simulink model "model_tmp_1p"  (R2015b)
settings: Solver=ode15s  StartTime=0.0  StopTime=T_sim  FixedStep=dt  RelTol=1e-3
PreLoadFcn:
  | setup_tmp_1p;
InitFcn:
  | setup_tmp_1p;
values from neighbouring files (symbols this model uses):
  A_act = [-100 0 0 0 0 -100 0 0 0 0 -100 0 ... (16 elements, 4x4)]    [CD_spline.mat]    (also in CL_spline.mat; setup.m = -100*eye(4); setup_tmp_1p.m = -100*eye(4); setup_tmp_4p.m = -100*eye(4))
  A_Kite = 7    [CD_spline.mat]    (also in CL_spline.mat; setup.m = 10.18; setup_tmp_1p.m = 10.18; setup_tmp_4p.m = 10.18)
  A_prd = [0 0 0 -640 0 0 0 0 0 0 -640 0 ... (36 elements, 6x6)]    [CD_spline.mat]    (also in CL_spline.mat; setup.m = 1000 * A_M_aug; setup_tmp_1p.m = 1000 * A_M_aug; setup_tmp_4p.m = 1000 * A_M_aug)
  A_ref = [0 0 0 -10000 0 0 0 0 0 0 -10000 0 ... (36 elements, 6x6)]    [CD_spline.mat]    (also in CL_spline.mat; setup.m = zeros(6); setup_tmp_1p.m = zeros(6); setup_tmp_4p.m = zeros(6))
  A_t_ref_cl = [0 0 0 -0.64 0 0 0 0 0 0 -0.64 0 ... (36 elements, 6x6)]    [CD_spline.mat]    (also in CL_spline.mat; setup.m = A_t_ref; setup_tmp_1p.m = A_t_ref; setup_tmp_4p.m = A_t_ref)
  ASideRel = 0    [CD_spline.mat]    (also in CL_spline.mat; setup.m; setup_tmp_1p.m; setup_tmp_4p.m)
  B_act = [100 0 0 0 0 100 0 0 0 0 100 0 ... (16 elements, 4x4)]    [CD_spline.mat]    (also in CL_spline.mat; setup.m = 100*eye(4); setup_tmp_1p.m = 100*eye(4); setup_tmp_4p.m = 100*eye(4))
  B_ref = [0 0 0 10000 0 0 0 0 0 0 10000 0 ... (18 elements, 6x3)]    [CD_spline.mat]    (also in CL_spline.mat; setup.m = zeros(6,3); setup_tmp_1p.m = zeros(6,3); setup_tmp_4p.m = zeros(6,3))
  B_t_ref_cl = [0 0 0 0.64 0 0 0 0 0 0 0.64 0 ... (18 elements, 6x3)]    [CD_spline.mat]    (also in CL_spline.mat)
  Bpbl = [0 0 0 1 0 0 0 0 0 0 1 0 ... (18 elements, 6x3)]    [CD_spline.mat]    (also in CL_spline.mat; setup.m = [zeros(3); eye(3)]; setup_tmp_1p.m = [zeros(3); eye(3)]; setup_tmp_4p.m = [zeros(3); eye(3)])
  c0 = 614000    [CD_spline.mat]    (also in CL_spline.mat; setup.m; setup_tmp_1p.m; setup_tmp_4p.m)
  C_A = [0 0.3 -1e-06 1 -0.3 0 1e-06 1 0 -0.3 -1e-06 1 ... (16 elements, 4x4)]    [CD_spline.mat]    (also in CL_spline.mat; setup.m = [0, -R, 0, R; setup_tmp_1p.m = [0, -R, 0, R; setup_tmp_4p.m = [0, -R, 0, R)
  C_A_inv = [0 -1.66666666667 -1.23358113847e-17 1.66666666667 1.66666666667 2.46716227694e-17 -1.66666666667 0 -250000 250000 -250000 250000 ... (16 elements, 4x4)]    [CD_spline.mat]    (also in CL_spline.mat; setup.m = C_A \eye(4); setup_tmp_1p.m = C_A \eye(4); setup_tmp_4p.m = C_A \eye(4))
  C_D_Kite = 0.05    [CD_spline.mat]    (also in CL_spline.mat; setup.m = 0.005; setup_tmp_1p.m = 0.005; setup_tmp_4p.m = 0.005)
  C_L_Kite = 0.1    [CD_spline.mat]    (also in CL_spline.mat; setup.m = 0.01; setup_tmp_1p.m = 0.01; setup_tmp_4p.m = 0.01)
  CD_tether = 0.96    [CD_spline.mat]    (also in CL_spline.mat; setup.m; setup_tmp_1p.m; setup_tmp_4p.m)
  d0 = 473    [CD_spline.mat]    (also in CL_spline.mat; setup.m; setup_tmp_1p.m; setup_tmp_4p.m)
  d_tether = 0.004    [CD_spline.mat]    (also in CL_spline.mat; setup.m; setup_tmp_1p.m; setup_tmp_4p.m)
  delta_dead = 0.5    [CD_spline.mat]    (also in CL_spline.mat; setup.m; setup_tmp_1p.m; setup_tmp_4p.m)
  e_0 = 0.01    [CD_spline.mat]    (also in CL_spline.mat; setup.m; setup_tmp_1p.m; setup_tmp_4p.m)
  epsilon = 0.6    [CD_spline.mat]    (also in CL_spline.mat; setup.m; setup_tmp_1p.m; setup_tmp_4p.m)
  eta_init = [0 0 0]    [CD_spline.mat]    (also in CL_spline.mat; setup.m = zeros(3,1); setup_tmp_1p.m = zeros(3,1); setup_tmp_4p.m = zeros(3,1))
  g = 9.81    [CD_spline.mat]    (also in CL_spline.mat; setup.m; setup_tmp_1p.m; setup_tmp_4p.m)
  g_vec = [0 0 9.81]    [CD_spline.mat]    (also in CL_spline.mat; setup.m = [0;0;9.81]; setup_tmp_1p.m = [0;0;9.81]; setup_tmp_4p.m = [0;0;9.81])
  Gamma_ad = 100    [CD_spline.mat]    (also in CL_spline.mat; setup.m = 100;100; setup_tmp_1p.m = 100;100; setup_tmp_4p.m = 100;100)
  Gamma_pred = 100    [CD_spline.mat]    (also in CL_spline.mat; setup.m; setup_tmp_1p.m; setup_tmp_4p.m)
  J = [0.018  0  0; 0  0.018  0; 0  0  0.009]    [CD_spline.mat]    (also in CL_spline.mat; setup.m = diag([Ixx, Iyy, Izz]); setup_tmp_1p.m = diag([Ixx, Iyy, Izz]); setup_tmp_4p.m = diag([Ixx, Iyy, Izz]))
  Jinv = [55.5555555556  0  0; 0  55.5555555556  0; 0  0  111.111111111]    [CD_spline.mat]    (also in CL_spline.mat; setup.m = J \ eye(3); setup_tmp_1p.m = J \ eye(3); setup_tmp_4p.m = J \ eye(3))
  k_e_eta = 10000    [CD_spline.mat]    (also in CL_spline.mat; setup.m; setup_tmp_1p.m; setup_tmp_4p.m)
  k_e_eta_dot = 400    [CD_spline.mat]    (also in CL_spline.mat; setup.m; setup_tmp_1p.m; setup_tmp_4p.m)
  k_e_eta_I = 1    [CD_spline.mat]    (also in CL_spline.mat; setup.m; setup_tmp_1p.m; setup_tmp_4p.m)
  K_i_t = [10  0  0; 0  10  0; 0  0  10]    [CD_spline.mat]    (also in CL_spline.mat; setup.m = 10*eye(3); setup_tmp_1p.m = 10*eye(3); setup_tmp_4p.m = 10*eye(3))
  K_v_t = [1.6  0  0; 0  1.6  0; 0  0  1.6]    [CD_spline.mat]    (also in CL_spline.mat; setup.m = 2*omega_0_trans*zeta_0_trans*eye(3); setup_tmp_1p.m = 2*omega_0_trans*zeta_0_trans*eye(3); setup_tmp_4p.m = 2*omega_0_trans*zeta_0_trans*eye(3))
  K_x_t = [0.64  0  0; 0  0.64  0; 0  0  0.64]    [CD_spline.mat]    (also in CL_spline.mat; setup.m = omega_0_trans^2*eye(3); setup_tmp_1p.m = omega_0_trans^2*eye(3); setup_tmp_4p.m = omega_0_trans^2*eye(3))
  l_s0 = 1    [CD_spline.mat]    (also in CL_spline.mat; setup.m = 1.42857142857; setup_tmp_1p.m = 1.42857142857; setup_tmp_4p.m = 2)
  m_kite = 7    [CD_spline.mat]    (also in CL_spline.mat; setup.m; setup_tmp_1p.m = 5;7; setup_tmp_4p.m = 6.21)
  m_p = 0.013    [CD_spline.mat]    (also in CL_spline.mat; setup.m = 0.0185714285714; setup_tmp_1p.m = 0.0185714285714; setup_tmp_4p.m = 0.026)
  m_uav = 3    [CD_spline.mat]    (also in CL_spline.mat; setup.m; setup_tmp_1p.m; setup_tmp_4p.m)
  n = 10    [CD_spline.mat]    (also in CL_spline.mat; setup.m; setup_tmp_1p.m; setup_tmp_4p.m)
  omega_init = [0 0 0]    [CD_spline.mat]    (also in CL_spline.mat; setup.m = zeros(3,1); setup_tmp_1p.m = zeros(3,1); setup_tmp_4p.m = zeros(3,1))
  p_init = [0 0 1 0 0 2 0 0 3 0 0 4 ... (30 elements, 30x1)]    [CD_spline.mat]    (also in CL_spline.mat; setup.m = zeros(3*n,1); setup_tmp_1p.m = zeros(3*n,1); setup_tmp_4p.m = zeros(3*n,1))
  P_prd = [712.5 0 0 156.25 0 0 0 712.5 0 0 156.25 0 ... (36 elements, 6x6)]    [CD_spline.mat]    (also in CL_spline.mat; setup.m = 1000 * P_tref; setup_tmp_1p.m = 1000 * P_tref; setup_tmp_4p.m = 1000 * P_tref)
  P_tref = [0.7125 0 0 0.15625 0 0 0 0.7125 0 0 0.15625 0 ... (36 elements, 6x6)]    [CD_spline.mat]    (also in CL_spline.mat; setup.m = lyap(A_M_aug', Q); setup_tmp_1p.m = lyap(A_M_aug', Q); setup_tmp_4p.m = lyap(A_M_aug', Q))
  rho_air = 1.225    [CD_spline.mat]    (also in CL_spline.mat; setup.m; setup_tmp_1p.m; setup_tmp_4p.m)
  rho_t = 0.013    [CD_spline.mat]    (also in CL_spline.mat; setup.m; setup_tmp_1p.m; setup_tmp_4p.m)
  sample_log = 0.01    [CD_spline.mat]    (also in CL_spline.mat; setup.m; setup_tmp_1p.m; setup_tmp_4p.m)
  t0 = 1    [CD_spline.mat]    (also in CL_spline.mat; setup.m; setup_tmp_1p.m; setup_tmp_4p.m)
  t1 = 3    [CD_spline.mat]    (also in CL_spline.mat; setup.m; setup_tmp_1p.m; setup_tmp_4p.m)
  T_launch = 40    [CD_spline.mat]    (also in CL_spline.mat; setup.m; setup_tmp_1p.m; setup_tmp_4p.m)
  Theta_max = 60    [CD_spline.mat]    (also in CL_spline.mat; setup.m; setup_tmp_1p.m; setup_tmp_4p.m)
  Thrust_Max = 80    [CD_spline.mat]    (also in CL_spline.mat; setup.m; setup_tmp_1p.m = 100; setup_tmp_4p.m = 1000000000)
  Tx = 10    [CD_spline.mat]    (also in CL_spline.mat; setup.m; setup_tmp_1p.m; setup_tmp_4p.m)
  Ty = 10    [CD_spline.mat]    (also in CL_spline.mat; setup.m; setup_tmp_1p.m; setup_tmp_4p.m)
  Tz = 10    [CD_spline.mat]    (also in CL_spline.mat; setup.m; setup_tmp_1p.m; setup_tmp_4p.m)
  v_w_vec = [1 1 1]    [CD_spline.mat]    (also in CL_spline.mat; setup.m = [1;0;0]; setup_tmp_1p.m = [1;0;0]; setup_tmp_4p.m = [1;0;0])
  x0num = 0    [CD_spline.mat]    (also in CL_spline.mat; polynomial_trajectory.m = double( solutions_x.x0 ))
  x1num = 0    [CD_spline.mat]    (also in CL_spline.mat; polynomial_trajectory.m = double( solutions_x.x1 ))
  x2num = 0    [CD_spline.mat]    (also in CL_spline.mat; polynomial_trajectory.m = double( solutions_x.x2 ))
  x3num = 0.05    [CD_spline.mat]    (also in CL_spline.mat; polynomial_trajectory.m = double( solutions_x.x3 ))
  x4num = -0.0075    [CD_spline.mat]    (also in CL_spline.mat; polynomial_trajectory.m = double( solutions_x.x4 ))
  x5num = 0.0003    [CD_spline.mat]    (also in CL_spline.mat; polynomial_trajectory.m = double( solutions_x.x5 ))
  x_drone_init = [0 0 10]    [CD_spline.mat]    (also in CL_spline.mat; setup.m = p_init(3*n-2:3*n); setup_KiteModel_4points.m = pos_UAV_init; setup_tmp_1p.m = p_init(3*n-2:3*n))
  xT = 5    [CD_spline.mat]    (also in CL_spline.mat; setup.m; setup_tmp_1p.m = 10; setup_tmp_4p.m = 10)
  y0num = 0    [CD_spline.mat]    (also in CL_spline.mat; polynomial_trajectory.m = double( solutions_y.y0 ))
  y1num = 0    [CD_spline.mat]    (also in CL_spline.mat; polynomial_trajectory.m = double( solutions_y.y1 ))
  y2num = 0    [CD_spline.mat]    (also in CL_spline.mat; polynomial_trajectory.m = double( solutions_y.y2 ))
  y3num = 0.1    [CD_spline.mat]    (also in CL_spline.mat; polynomial_trajectory.m = double( solutions_y.y3 ))
  y4num = -0.015    [CD_spline.mat]    (also in CL_spline.mat; polynomial_trajectory.m = double( solutions_y.y4 ))
  y5num = 0.0006    [CD_spline.mat]    (also in CL_spline.mat; polynomial_trajectory.m = double( solutions_y.y5 ))
  yT = 10    [CD_spline.mat]    (also in CL_spline.mat; setup.m; setup_tmp_1p.m = 0; setup_tmp_4p.m = 0)
  z0num = 10    [CD_spline.mat]    (also in CL_spline.mat; polynomial_trajectory.m = double( solutions_z.z0 ))
  z1num = 0    [CD_spline.mat]    (also in CL_spline.mat; polynomial_trajectory.m = double( solutions_z.z1 ))
  z2num = 0    [CD_spline.mat]    (also in CL_spline.mat; polynomial_trajectory.m = double( solutions_z.z2 ))
  z3num = 0.4    [CD_spline.mat]    (also in CL_spline.mat; polynomial_trajectory.m = double( solutions_z.z3 ))
  z4num = -0.06    [CD_spline.mat]    (also in CL_spline.mat; polynomial_trajectory.m = double( solutions_z.z4 ))
  z5num = 0.0024    [CD_spline.mat]    (also in CL_spline.mat; polynomial_trajectory.m = double( solutions_z.z5 ))
  zT = 50    [CD_spline.mat]    (also in CL_spline.mat; setup.m; setup_tmp_1p.m; setup_tmp_4p.m)
libraries: simulink x1
(part 2 of 2)

== system model_tmp_1p/Controller/Outer_Loop_Position/Adaptive_Augmentation/Proj(Theta_hat, GammaY)_1column ==
  note: Ref.: Lavretsky, Robust and Adaptive Control, p. 329
      | Lecure Notes Nonlinear and Adaptive Control, TU Munich, FSD, SS2014, Robustness Modifications
  Theta_hat : Inport
  Theta_dot : Inport  Port=2
  Mux : Mux  Inputs=3
  Proj(Theta,Theta_dot) : MATLAB Function  TreatAsAtomicUnit=on
  Reshape1 : Reshape  OutputDimensionality=Row vector (2-D)
  Reshape2 : Reshape  OutputDimensionality=Row vector (2-D)
  To Workspace1 : ToWorkspace  VariableName=proj_flat  SaveFormat=Timeseries  SampleTime=sample_log
      settings: Save2DSignal=2-D array (concatenate along first dimension)
  To Workspace2 : ToWorkspace  VariableName=Theta_dot_save  SampleTime=sample_log
      settings: Save2DSignal=2-D array (concatenate along first dimension)
  To Workspace3 : ToWorkspace  VariableName=orthogonal_part  SampleTime=sample_log
      settings: Save2DSignal=2-D array (concatenate along first dimension)
  calculate_f : MATLAB Function  TreatAsAtomicUnit=on
  calculate_gradf : MATLAB Function  TreatAsAtomicUnit=on
  max_allowable_bound : Constant  Value=Theta_max
  projection_tolerance : Constant  Value=epsilon
  Theta_hat_dot : Outport
  wires:
  Proj(Theta,Theta_dot)/2(Theta_hat_dot_) -> Reshape1/1, Theta_hat_dot/1
  Proj(Theta,Theta_dot)/1(flag) -> Mux/2
  Proj(Theta,Theta_dot)/3(direction) -> Mux/3
  Mux/1 -> To Workspace1/1
  calculate_gradf/1(gradf) -> Proj(Theta,Theta_dot)/2(gradf)
  Theta_hat/1 -> calculate_gradf/1(theta_hat), calculate_f/1(theta_hat)
  projection_tolerance/1 -> calculate_f/3(epsilon), calculate_gradf/3(epsilon)
  max_allowable_bound/1 -> calculate_f/2(Theta_max), calculate_gradf/2(Theta_max)
  Theta_dot/1 -> Proj(Theta,Theta_dot)/3(Theta_dot)
  calculate_f/1(f) -> Mux/1, Proj(Theta,Theta_dot)/1(f)
  Reshape1/1 -> To Workspace2/1
  Proj(Theta,Theta_dot)/4(orthogonal_part) -> Reshape2/1
  Reshape2/1 -> To Workspace3/1

== system model_tmp_1p/Controller/Outer_Loop_Position/Adaptive_Augmentation/Proj(Theta_hat, GammaY)_multicolumns ==
  note: Ref.: Lavretsky, Robust and Adaptive Control, p. 329
      | Lecure Notes Nonlinear and Adaptive Control, TU Munich, FSD, SS2014, Robustness Modifications
  Theta_hat : Inport
  Theta_dot : Inport  Port=2
  MATLAB Function : MATLAB Function  TreatAsAtomicUnit=on
  Matrix Concatenate : Concatenate  NumInputs=3  Mode=Multidimensional array
  Projection_Input_1 : Subsystem
  Projection_Input_2 : Subsystem
  Projection_Input_3 : Subsystem
  Theta_hat_dot : Outport
  wires:
  Theta_hat/1 -> MATLAB Function/1(Theta_hat)
  Theta_dot/1 -> MATLAB Function/2(Theta_hat_dot)
  Projection_Input_1/1(Out1) -> Matrix Concatenate/1
  MATLAB Function/1(Theta_hat_1) -> Projection_Input_1/1(In1)
  MATLAB Function/2(Theta_hat_dot_1) -> Projection_Input_1/2(In2)
  MATLAB Function/3(Theta_hat_2) -> Projection_Input_2/1(In1)
  MATLAB Function/4(Theta_hat_dot_2) -> Projection_Input_2/2(In2)
  MATLAB Function/6(Theta_hat_dot_3) -> Projection_Input_3/2(In2)
  MATLAB Function/5(Theta_hat_3) -> Projection_Input_3/1(In1)
  Projection_Input_2/1(Out1) -> Matrix Concatenate/2
  Projection_Input_3/1(Out1) -> Matrix Concatenate/3
  Matrix Concatenate/1 -> Theta_hat_dot/1

== system model_tmp_1p/Controller/Outer_Loop_Position/Adaptive_Augmentation/Smooth_Deadzone_MRAC ==
  note: Ref.: Lavretsky, Robust and Adaptive Control, p. 319
  e : Inport
  Dead_Zone_Mod1 : Constant  Value=delta_dead
  Dead_Zone_Mod2 : Constant  Value=e_0
  Dot Product : DotProduct  InputSameDT=on  OutDataTypeStr=Inherit: Inherit via internal rule
  Mux : Mux  Inputs=2
  Sqrt : Sqrt  SaturateOnIntegerOverflow=on
  To Workspace8 : ToWorkspace  VariableName=e_ref_mu  SaveFormat=Timeseries  SampleTime=sample_log
      settings: Save2DSignal=2-D array (concatenate along first dimension)
  smooth_deadzone : MATLAB Function  TreatAsAtomicUnit=on
  mu_dead : Outport
  wires:
  e/1 -> Dot Product/1, Dot Product/2
  Dead_Zone_Mod1/1 -> smooth_deadzone/2(delta_dead)
  Dead_Zone_Mod2/1 -> smooth_deadzone/3(e_0)
  Dot Product/1 -> Sqrt/1
  Sqrt/1 -> Mux/1, smooth_deadzone/1(e_norm)
  smooth_deadzone/1(mu_dead) -> Mux/2, mu_dead/1
  Mux/1 -> To Workspace8/1

== system model_tmp_1p/Controller/Outer_Loop_Position/Adaptive_Augmentation/Smooth_Deadzone_PMRAC ==
  note: Ref.: Lavretsky, Robust and Adaptive Control, p. 319
  e : Inport
  Dead_Zone_Mod1 : Constant  Value=delta_dead
  Dead_Zone_Mod2 : Constant  Value=e_0
  Dot Product : DotProduct  InputSameDT=on  OutDataTypeStr=Inherit: Inherit via internal rule
  Mux1 : Mux  Inputs=2
  Sqrt : Sqrt  SaturateOnIntegerOverflow=on
  To Workspace1 : ToWorkspace  VariableName=e_pref_mu  SaveFormat=Timeseries  SampleTime=sample_log
      settings: Save2DSignal=2-D array (concatenate along first dimension)
  smooth_deadzone : MATLAB Function  TreatAsAtomicUnit=on
  mu_dead : Outport
  wires:
  Dot Product/1 -> Sqrt/1
  Dead_Zone_Mod2/1 -> smooth_deadzone/3(e_0)
  Dead_Zone_Mod1/1 -> smooth_deadzone/2(delta_dead)
  e/1 -> Dot Product/2, Dot Product/1
  Sqrt/1 -> Mux1/1, smooth_deadzone/1(e_norm)
  smooth_deadzone/1(mu_dead) -> Mux1/2, mu_dead/1
  Mux1/1 -> To Workspace1/1

== system model_tmp_1p/Plant/Tether_Kite_Tether_UAV_Dynamics_1P/First_order_lag_Actuator/Actuator ==
  Propeller_RPMs_cmd : Inport
  Add : Sum  Inputs=+-
  Gain : Gain  Gain=B_act  Multiplication=Matrix(K*u)
  Gain1 : Gain  Gain=A_act  Multiplication=Matrix(K*u)
  Integrator Limited1 : Integrator  InitialCondition=zeros(4,1)  LimitOutput=on  UpperSaturationLimit=Thrust_Max  LowerSaturationLimit=-Thrust_Max
  Output_Actuator : Gain  Gain=C_A  Multiplication=Matrix(K*u)
  Reaction_Deficit_Actuators : Scope
  Sum : Sum  Inputs=|++
  To Workspace1 : ToWorkspace  VariableName=prop_thrust_cmd  SaveFormat=Timeseries  SampleTime=sample_log
  To Workspace2 : ToWorkspace  VariableName=prop_thrust_real  SaveFormat=Timeseries  SampleTime=sample_log
  Thrust_Moments : Outport
  wires:
  Output_Actuator/1 -> Thrust_Moments/1
  Gain/1 -> Sum/1
  Gain1/1 -> Sum/2
  Sum/1 -> Integrator Limited1/1
  Propeller_RPMs_cmd/1 -> Add/1, To Workspace1/1, Gain/1
  Add/1 -> Reaction_Deficit_Actuators/1
  Integrator Limited1/1 -> Add/2, To Workspace2/1, Gain1/1, Output_Actuator/1

== system model_tmp_1p/Controller/Outer_Loop_Position/Adaptive_Augmentation/Proj(Theta_hat, GammaY)_multicolumns/Projection_Input_1 ==
  In1 : Inport
  In2 : Inport  Port=2
  Proj(Theta,Theta_dot) : MATLAB Function  TreatAsAtomicUnit=on
  calculate_f : MATLAB Function  TreatAsAtomicUnit=on
  calculate_gradf : MATLAB Function  TreatAsAtomicUnit=on
  max_allowable_bound : Constant  Value=Theta_max
  projection_tolerance : Constant  Value=epsilon
  Out1 : Outport
  wires:
  calculate_f/1(f) -> Proj(Theta,Theta_dot)/1(f)
  In2/1 -> Proj(Theta,Theta_dot)/3(Theta_dot)
  max_allowable_bound/1 -> calculate_f/2(Theta_max), calculate_gradf/2(Theta_max)
  projection_tolerance/1 -> calculate_f/3(epsilon), calculate_gradf/3(epsilon)
  In1/1 -> calculate_gradf/1(theta_hat), calculate_f/1(theta_hat)
  calculate_gradf/1(gradf) -> Proj(Theta,Theta_dot)/2(gradf)
  Proj(Theta,Theta_dot)/1(Theta_hat_dot_) -> Out1/1

== system model_tmp_1p/Controller/Outer_Loop_Position/Adaptive_Augmentation/Proj(Theta_hat, GammaY)_multicolumns/Projection_Input_2 ==
  In1 : Inport
  In2 : Inport  Port=2
  Proj(Theta,Theta_dot) : MATLAB Function  TreatAsAtomicUnit=on
  calculate_f : MATLAB Function  TreatAsAtomicUnit=on
  calculate_gradf : MATLAB Function  TreatAsAtomicUnit=on
  max_allowable_bound : Constant  Value=Theta_max
  projection_tolerance : Constant  Value=epsilon
  Out1 : Outport
  wires:
  calculate_f/1(f) -> Proj(Theta,Theta_dot)/1(f)
  In2/1 -> Proj(Theta,Theta_dot)/3(Theta_dot)
  max_allowable_bound/1 -> calculate_f/2(Theta_max), calculate_gradf/2(Theta_max)
  projection_tolerance/1 -> calculate_f/3(epsilon), calculate_gradf/3(epsilon)
  In1/1 -> calculate_gradf/1(theta_hat), calculate_f/1(theta_hat)
  calculate_gradf/1(gradf) -> Proj(Theta,Theta_dot)/2(gradf)
  Proj(Theta,Theta_dot)/1(Theta_hat_dot_) -> Out1/1

== system model_tmp_1p/Controller/Outer_Loop_Position/Adaptive_Augmentation/Proj(Theta_hat, GammaY)_multicolumns/Projection_Input_3 ==
  In1 : Inport
  In2 : Inport  Port=2
  Mux : Mux  Inputs=3
  Proj(Theta,Theta_dot) : MATLAB Function  TreatAsAtomicUnit=on
  Scope : Scope
  Scope1 : Scope
  To Workspace1 : ToWorkspace  VariableName=proj_flat  SaveFormat=Timeseries  SampleTime=sample_log
      settings: Save2DSignal=2-D array (concatenate along first dimension)
  calculate_f : MATLAB Function  TreatAsAtomicUnit=on
  calculate_gradf : MATLAB Function  TreatAsAtomicUnit=on
  max_allowable_bound : Constant  Value=Theta_max
  projection_tolerance : Constant  Value=epsilon
  Out1 : Outport
  wires:
  calculate_f/1(f) -> Mux/1, Proj(Theta,Theta_dot)/1(f)
  In2/1 -> Proj(Theta,Theta_dot)/3(Theta_dot)
  max_allowable_bound/1 -> calculate_f/2(Theta_max), calculate_gradf/2(Theta_max)
  projection_tolerance/1 -> calculate_f/3(epsilon), calculate_gradf/3(epsilon)
  In1/1 -> calculate_gradf/1(theta_hat), calculate_f/1(theta_hat)
  calculate_gradf/1(gradf) -> Proj(Theta,Theta_dot)/2(gradf)
  Proj(Theta,Theta_dot)/2(Theta_hat_dot_) -> Out1/1
  Mux/1 -> To Workspace1/1
  Proj(Theta,Theta_dot)/3(direction) -> Scope/1, Mux/3
  Proj(Theta,Theta_dot)/1(flag) -> Scope1/1, Mux/2

== matlab function model_tmp_1p/Controller/Inner_Loop_Attitude/Plant_Inversion_RD2/Plant_Inversion ==
  data: omega input; u_NDI output; eta input; eta_dot input; J input; nu_tot input
function u_NDI = fcn(omega, eta, eta_dot, J, nu_tot)
%#codegen
p = omega(1); 
q = omega(2); 
r = omega(3); 
Ix = J(1,1); 
Iy = J(2,2); 
Iz = J(3,3); 


cross_coupling = [ Iy*q*r - Iz*q*r
 Iz*p*r - Ix*p*r;
 Ix*p*q - Iy*p*q];

% T_inv = [1, sin(eta(1)) * tan(eta(2)), cos(eta(1)) * tan(eta(2)) ; 
% 0, cos(eta(1)), -sin(eta(1)); 
% 0, sin(eta(1))/cos(eta(2)), cos(eta(1))/cos(eta(2))] \ eye(3); 

T_inv = [1, 0, -sin(eta(2));
         0, cos(eta(1)), sin(eta(1))*cos(eta(2));
         0, -sin(eta(1)), cos(eta(1))*cos(eta(2))];
     
T_dot = eta_dot(1) * [0, cos(eta(1)) * tan(eta(2)), -sin(eta(1))*tan(eta(2)); 
                      0, -sin(eta(1)), -cos(eta(1));
                      0, cos(eta(1))/cos(eta(2)), -sin(eta(1))/cos(eta(2))]+...
        eta_dot(2) * [0, sin(eta(1))/cos(eta(2))^2, cos(eta(1))/cos(eta(2))^2; 
                       0, 0, 0; 
                       0, sin(eta(1))*sin(eta(2))/cos(eta(2))^2, cos(eta(1))*sin(eta(2))/cos(eta(2))^2];
                          
u_NDI = -cross_coupling + J * T_inv * ( -T_dot * omega + nu_tot);

== matlab function model_tmp_1p/Flight_Path_Planner/Reference_Dynamic_x1 ==
  data: t input; y_ref output; y0num parameter; y1num parameter; y2num parameter; y3num parameter; y4num parameter; y5num parameter; yT parameter; Ty parameter
function y_ref = fcn(t,y0num, y1num, y2num, y3num, y4num, y5num, yT,Ty )

if t >= Ty
    y_ref = yT;
else
    y_ref = y5num * t^5 + y4num * t^4 + y3num * t^3 + y2num * t^2 + y1num * t + y0num;
end

== matlab function model_tmp_1p/Flight_Path_Planner/Reference_Dynamic_x3 ==
  data: t input; x_ref output; x0num parameter; x1num parameter; x2num parameter; x3num parameter; x4num parameter; x5num parameter; Tx parameter; xT parameter
function x_ref = fcn(t,x0num, x1num, x2num, x3num, x4num, x5num, Tx,xT )

if t >= Tx
    x_ref = xT;
else
    x_ref = x5num * t^5 + x4num * t^4 + x3num * t^3 + x2num * t^2 + x1num * t + x0num;
end

== matlab function model_tmp_1p/Flight_Path_Planner2/Reference_Dynamic_x ==
  data: x_cmd input; x_ref input; x_ref_dot output; t0 parameter; t1 parameter
function x_ref_dot = fcn(x_cmd, x_ref, t0, t1)

% a0 = 1;
% a1 = 5;

x_ref_dot = [0,1;
                -t0, -t1]*x_ref + [0;t0] * x_cmd;

== matlab function model_tmp_1p/Controller/Inner_Loop_Attitude/estimate_eta_dot ==
  data: omega input; eta input; eta_dot output
function eta_dot  = fcn( omega, eta)
%#codegen

eta_dot = [1, sin(eta(1)) * tan(eta(2)), cos(eta(1)) * tan(eta(2)) ; 
0, cos(eta(1)), -sin(eta(1)); 
0, sin(eta(1))/cos(eta(2)), cos(eta(1))/cos(eta(2))] * omega;

== matlab function model_tmp_1p/Flight_Path_Planner/Reference_Dynamic_x2 ==
  data: t input; z_ref output; z0num parameter; z1num parameter; z2num parameter; z3num parameter; z4num parameter; z5num parameter; Tz parameter; zT parameter
function z_ref = fcn(t,z0num, z1num, z2num, z3num, z4num, z5num,Tz, zT)

if t >= Tz
    z_ref = zT;
else
    z_ref = z5num * t^5 + z4num * t^4 + z3num * t^3 + z2num * t^2 + z1num * t + z0num;
end

== matlab function model_tmp_1p/Controller/Outer_Loop_Position/Adaptive_Augmentation/Smooth_Deadzone_PMRAC/smooth_deadzone ==
  data: e_norm input; mu_dead output; delta_dead input; e_0 input
function mu_dead = fcn(e_norm, delta_dead, e_0)
%#codegen

mu_dead = max( 0, min( 1, (e_norm - delta_dead*e_0)/...
                          ( (1-delta_dead) * e_0) ) );

== matlab function model_tmp_1p/Controller/Outer_Loop_Position/Predictor_Model_Translational_Dynamics/Reference_Model_Position ==
  data: A_prd input; A_ref input; x_prd_dotdot output; B_ref input; x_cmd input; x_p input; x_prd input
function x_prd_dotdot  = fcn(A_prd,A_ref,B_ref, x_cmd,x_p,x_prd)

    x_prd_dotdot = A_prd * (x_prd - x_p) + A_ref * x_p + B_ref * x_cmd;

== matlab function model_tmp_1p/Controller/Outer_Loop_Position/Reference_Model_Translational_Dynamics/Reference_Model_Position ==
  data: A_t_ref_cl input; x_ref_dotdot output; B_t_ref input; x_cmd input; x_ref input
function x_ref_dotdot  = fcn(A_t_ref_cl,B_t_ref, x_cmd,x_ref)

    x_ref_dotdot = A_t_ref_cl * x_ref + B_t_ref * x_cmd;

== matlab function model_tmp_1p/Controller/Outer_Loop_Position/Adaptive_Augmentation/Proj(Theta_hat, GammaY)_multicolumns/MATLAB Function ==
  data: Theta_hat input; Theta_hat_1 output; Theta_hat_dot_1 output; Theta_hat_dot input; Theta_hat_2 output; Theta_hat_dot_2 output; Theta_hat_3 output; Theta_hat_dot_3 output
function [Theta_hat_1,Theta_hat_dot_1, Theta_hat_2, Theta_hat_dot_2,...
            Theta_hat_3, Theta_hat_dot_3] = fcn(Theta_hat, Theta_hat_dot)
%#codegen
Theta_hat_1 = Theta_hat(1,:);
Theta_hat_2 = Theta_hat(2,:);
Theta_hat_3 = Theta_hat(3,:);

Theta_hat_dot_1 = Theta_hat_dot(1,:); 
Theta_hat_dot_2 = Theta_hat_dot(2,:);
Theta_hat_dot_3 = Theta_hat_dot(3,:);

== matlab function model_tmp_1p/Controller/Outer_Loop_Position/Adaptive_Augmentation/Proj(Theta_hat, GammaY)_multicolumns/Projection_Input_1/Proj(Theta,Theta_dot) ==
  data: f input; gradf input; Theta_dot input; Theta_hat_dot_ output
function  Theta_hat_dot_ = fcn(f, gradf, Theta_dot )
%#codegen


if ( f > 0 && gradf*Theta_dot' > 0 )
    Theta_hat_dot_ = Theta_dot - f * ( (gradf'*gradf) / (gradf*gradf') * Theta_dot' )'   ;
else
    Theta_hat_dot_ =  Theta_dot;
end

== matlab function model_tmp_1p/Controller/Outer_Loop_Position/Total_Thrust ==
  data: T_ref input; T_tot output
function T_tot  = fcn(T_ref)

%T_z = [0;0;norm(T_ref)];
T_tot = norm(T_ref);

== matlab function model_tmp_1p/Controller/Outer_Loop_Position/Adaptive_Augmentation/Proj(Theta_hat, GammaY)_multicolumns/Projection_Input_1/calculate_f ==
  data: theta_hat input; f output; Theta_max input; epsilon input
function f   = fcn(theta_hat,Theta_max, epsilon )
%#codegen
f = ( (1+epsilon)*norm(theta_hat)^2 - (Theta_max)^2 ) / (epsilon*(Theta_max)^2);

== matlab function model_tmp_1p/Controller/Outer_Loop_Position/Adaptive_Augmentation/Proj(Theta_hat, GammaY)_multicolumns/Projection_Input_1/calculate_gradf ==
  data: theta_hat input; gradf output; Theta_max input; epsilon input
function gradf = fcn(theta_hat,Theta_max, epsilon )
%#codegen
gradf = ( 2*(1+epsilon) ) / (epsilon*(Theta_max)^2) * theta_hat ;

== matlab function model_tmp_1p/Controller/Pseudo_Control_Hedging/Rotate thrust vector according to attitude ==
  data: u_Thrust_I input; eta input; u_Thrust_B output
function u_Thrust_B   = thrust_Bz_direction(  u_Thrust_I, eta) 

phi = eta(1); 
theta = eta(2); 
psi = eta(3); 

% Rotate thrust vector such that it is perpendicular to the "rotor blades"
u_Thrust_B = [cos(psi)*cos(theta), sin(psi)*cos(theta), -sin(theta); 
            cos(psi)*sin(theta)*sin(phi)-sin(psi)*cos(phi), sin(psi)*sin(theta)*sin(phi)+cos(psi)*cos(phi), cos(theta)*sin(phi); 
            cos(psi)*sin(theta)*cos(phi)+sin(psi)*sin(phi), sin(psi)*sin(theta)*cos(phi)-cos(psi)*sin(phi), cos(theta)*cos(phi)] *...
            [0;0;u_Thrust_I];

== matlab function model_tmp_1p/Controller/Pseudo_Control_Hedging/Plant_Inversion_RD2_backwards/Plant_Inversion ==
  data: omega input; nu_tot_rot_hat output; eta input; eta_dot input; J parameter; Jinv parameter; M_hat input
function nu_tot_rot_hat = fcn(omega, eta, eta_dot,J, Jinv, M_hat)
%#codegen
p = omega(1); 
q = omega(2); 
r = omega(3); 
Ix = J(1,1); 
Iy = J(2,2); 
Iz = J(3,3); 


cross_coupling = [ Iy*q*r - Iz*q*r
 Iz*p*r - Ix*p*r;
 Ix*p*q - Iy*p*q];

% T_inv = [1, sin(eta(1)) * tan(eta(2)), cos(eta(1)) * tan(eta(2)) ; 
% 0, cos(eta(1)), -sin(eta(1)); 
% 0, sin(eta(1))/cos(eta(2)), cos(eta(1))/cos(eta(2))] \ eye(3); 

T = [1, sin(eta(1)) * tan(eta(2)), cos(eta(1)) * tan(eta(2)) ; 
0, cos(eta(1)), -sin(eta(1)); 
0, sin(eta(1))/cos(eta(2)), cos(eta(1))/cos(eta(2))];

T_dot = eta_dot(1) * [0, cos(eta(1)) * tan(eta(2)), -sin(eta(1))*tan(eta(2)); 
                      0, -sin(eta(1)), -cos(eta(1));
                      0, cos(eta(1))/cos(eta(2)), -sin(eta(1))/cos(eta(2))]+...
        eta_dot(2) * [0, sin(eta(1))/cos(eta(2))^2, cos(eta(1))/cos(eta(2))^2; 
                       0, 0, 0; 
                       0, sin(eta(1))*sin(eta(2))/cos(eta(2))^2, cos(eta(1))*sin(eta(2))/cos(eta(2))^2];
                          
%u_NDI = -cross_coupling + J * T_inv * ( -T_dot * omega + nu_tot); 

nu_tot_rot_hat = T * Jinv * ( M_hat + cross_coupling ) + T_dot *omega;

== matlab function model_tmp_1p/Controller/Pseudo_Control_Hedging/Plant_Inversion_RD2_backwards/estimate_eta_dot ==
  data: omega input; eta input; eta_dot output
function eta_dot  = fcn( omega, eta)
%#codegen

eta_dot = [1, sin(eta(1)) * tan(eta(2)), cos(eta(1)) * tan(eta(2)) ; 
0, cos(eta(1)), -sin(eta(1)); 
0, sin(eta(1))/cos(eta(2)), cos(eta(1))/cos(eta(2))] * omega;

== matlab function model_tmp_1p/Controller/Outer_Loop_Position/Adaptive_Augmentation/Smooth_Deadzone_MRAC/smooth_deadzone ==
  data: e_norm input; mu_dead output; delta_dead input; e_0 input
function mu_dead = fcn(e_norm, delta_dead, e_0)
%#codegen

mu_dead = max( 0, min( 1, (e_norm - delta_dead*e_0)/...
                          ( (1-delta_dead) * e_0) ) );

== matlab function model_tmp_1p/Controller/Outer_Loop_Position/Calc_Ref_Attitude ==
  data: T_ref input; Eta_Cmd output; eta input
function Eta_Cmd  = fcn(T_ref, eta)
%#codegen
psi = eta(3); 
theta = eta(2); 
phi = eta(1); 

psi_c = 0;

T = norm( T_ref ); 

phi_c = -asin( 1/T * (T_ref(1) * sin(psi_c) - T_ref(2) * cos(psi_c)) ); 
theta_c = -atan( 1/T_ref(3) * (T_ref(1) * cos(psi_c) + T_ref(2) * sin(psi_c))); 

Eta_Cmd = [phi_c;theta_c; 0];

== matlab function model_tmp_1p/Plant/Tether_Kite_Tether_UAV_Dynamics_1P/Kite_Model_1P/Kite_Model ==
  data: launch_flag input; x_dotdot_kite output; rho_air parameter; A_Kite parameter; g_vec parameter; C_L_Kite parameter; C_D_Kite parameter; m_kite parameter; v_w_vec input; ASideRel parameter; xp_aboveKite input; x_kite input; xp_belowKite input; xdot_aboveKite input; xdot_kite input; xdot_belowKite input; l_s input; c0 parameter; d0 parameter; l_s0 parameter
function x_dotdot_kite  = fcn(launch_flag,...
    rho_air, A_Kite, g_vec, C_L_Kite, C_D_Kite, m_kite, v_w_vec, ASideRel,...
    xp_aboveKite, x_kite, xp_belowKite,xdot_aboveKite, xdot_kite,...
    xdot_belowKite, l_s, c0, d0, l_s0)

c = c0/l_s;
d = d0/l_s;

% Tether forces from below and above
f_T_below = calcSpringDamperForce(c, norm(x_kite-xp_belowKite) , l_s, d, x_kite - xp_belowKite, xdot_kite - xdot_belowKite, 1 );
f_T_above = calcSpringDamperForce(c0, norm(xp_aboveKite-x_kite), l_s0, d0, xp_aboveKite-x_kite, xdot_aboveKite - xdot_kite, 1 );

% Calculate the apparent wind speed
v_a_k = v_w_vec - xdot_kite;
if launch_flag
    C_L_Kite = 0.5;
    C_D_Kite = 0.2;
end

[L_kite, D_kite, S_kite] = calcKiteForces(x_kite, xp_belowKite, ...
                                        v_a_k, C_L_Kite, rho_air, A_Kite, C_D_Kite, ASideRel);
if launch_flag % kite is launched
    x_dotdot_kite = 1/m_kite * ( -f_T_below  - m_kite*g_vec  ... % remove the conection to 'drone tether'
        + D_kite + L_kite + 0*S_kite ) ;  % Kite dynamics
else
    x_dotdot_kite = 1/m_kite * ( -f_T_below + f_T_above - m_kite*g_vec  ...
        + 0*D_kite + 0*L_kite  + 0*S_kite);  % Kite dynamics
end

== matlab function model_tmp_1p/Controller/Outer_Loop_Position/Adaptive_Augmentation/Proj(Theta_hat, GammaY)_1column/Proj(Theta,Theta_dot) ==
  data: flag output; f input; gradf input; Theta_dot input; Theta_hat_dot_ output; direction output; orthogonal_part output
function  [flag,Theta_hat_dot_, direction, orthogonal_part] = fcn(f, gradf, Theta_dot )
%#codegen


if ( f > 0 && Theta_dot'*gradf > 0 )
    flag  = 1;
    direction = Theta_dot'*gradf;
    Theta_hat_dot_ = Theta_dot - f * ( (gradf*gradf') / (gradf'*gradf) * Theta_dot )   ;
    orthogonal_part = f * ( (gradf*gradf') / (gradf'*gradf) * Theta_dot );
else
    direction = Theta_dot'*gradf;
    flag = 0;
    Theta_hat_dot_ =  Theta_dot;
    orthogonal_part = zeros(3,1);
end

== matlab function model_tmp_1p/Controller/Outer_Loop_Position/Adaptive_Augmentation/Proj(Theta_hat, GammaY)_1column/calculate_f ==
  data: theta_hat input; f output; Theta_max input; epsilon input
function f   = fcn(theta_hat,Theta_max, epsilon )
%#codegen
f = ( (1+epsilon)*norm(theta_hat)^2 - (Theta_max)^2 ) / (epsilon*(Theta_max)^2);

== matlab function model_tmp_1p/Controller/Outer_Loop_Position/Adaptive_Augmentation/Proj(Theta_hat, GammaY)_1column/calculate_gradf ==
  data: theta_hat input; gradf output; Theta_max input; epsilon input
function gradf = fcn(theta_hat,Theta_max, epsilon )
%#codegen
gradf = ( 2*(1+epsilon) ) / (epsilon*(Theta_max)^2) * theta_hat ;

== matlab function model_tmp_1p/Controller/Reelout_Speed_Control/Activation_Function ==
  data: d input; safety_factor_vro output
function safety_factor_vro = fcn(d)
%#codegen
zero_cross = 0.5;
% Sigmoid like function. Converges against 1 if d > zero_cross
% and against -1 if d < zero_cross. It is used to ensure that the 
% current tether length cannot enter the "safety-ball" around the drone.
safety_factor_vro = 2*( 1 ./ ( 1 + exp(-5*( d - zero_cross ) ) ) - 0.5 ) ;

== matlab function model_tmp_1p/Analysis/Evaluate_Lyapunovfunction ==
  data: xi input; V output; P input; d_hat input; gamma_d input; e_pred input; P_pred input; d_real input
function V = fcn(xi, P, d_hat, gamma_d, e_pred, P_pred,d_real)
%#codegen
d_real = [5;5;5];
d_tilde = -d_hat - d_real;
V = 0.5 * xi' * P * xi + ...
    0.5 * e_pred * P_pred * e_pred' + ...
    0.5 * trace(d_tilde * 1 / gamma_d * d_tilde');

== matlab function model_tmp_1p/Controller/Outer_Loop_Position/Adaptive_Augmentation/Proj(Theta_hat, GammaY)_multicolumns/Projection_Input_2/Proj(Theta,Theta_dot) ==
  data: f input; gradf input; Theta_dot input; Theta_hat_dot_ output
function  Theta_hat_dot_ = fcn(f, gradf, Theta_dot )
%#codegen


if ( f > 0 && gradf*Theta_dot' > 0 )
    Theta_hat_dot_ = Theta_dot - f * ( (gradf'*gradf) / (gradf*gradf') * Theta_dot' )'   ;
else
    Theta_hat_dot_ =  Theta_dot;
end

== matlab function model_tmp_1p/Controller/Outer_Loop_Position/Adaptive_Augmentation/Proj(Theta_hat, GammaY)_multicolumns/Projection_Input_2/calculate_f ==
  data: theta_hat input; f output; Theta_max input; epsilon input
function f   = fcn(theta_hat,Theta_max, epsilon )
%#codegen
f = ( (1+epsilon)*norm(theta_hat)^2 - (Theta_max)^2 ) / (epsilon*(Theta_max)^2);

== matlab function model_tmp_1p/Controller/Outer_Loop_Position/Adaptive_Augmentation/Proj(Theta_hat, GammaY)_multicolumns/Projection_Input_2/calculate_gradf ==
  data: theta_hat input; gradf output; Theta_max input; epsilon input
function gradf = fcn(theta_hat,Theta_max, epsilon )
%#codegen
gradf = ( 2*(1+epsilon) ) / (epsilon*(Theta_max)^2) * theta_hat ;

== matlab function model_tmp_1p/Controller/Outer_Loop_Position/Adaptive_Augmentation/Proj(Theta_hat, GammaY)_multicolumns/Projection_Input_3/Proj(Theta,Theta_dot) ==
  data: flag output; f input; gradf input; Theta_dot input; Theta_hat_dot_ output; direction output
function  [flag,Theta_hat_dot_, direction] = fcn(f, gradf, Theta_dot )
%#codegen


if ( f > 0 && gradf*Theta_dot' > 0 )
    flag  = 1;
    direction = gradf*Theta_dot';
    Theta_hat_dot_ = Theta_dot - f * ( (gradf'*gradf) / (gradf*gradf') * Theta_dot' )'   ;
else
    direction = gradf*Theta_dot';
    flag = 0;
    Theta_hat_dot_ =  Theta_dot;
end

== matlab function model_tmp_1p/Controller/Outer_Loop_Position/Adaptive_Augmentation/Proj(Theta_hat, GammaY)_multicolumns/Projection_Input_3/calculate_f ==
  data: theta_hat input; f output; Theta_max input; epsilon input
function f   = fcn(theta_hat,Theta_max, epsilon )
%#codegen
f = ( (1+epsilon)*norm(theta_hat)^2 - (Theta_max)^2 ) / (epsilon*(Theta_max)^2);

== matlab function model_tmp_1p/Controller/Outer_Loop_Position/Adaptive_Augmentation/Proj(Theta_hat, GammaY)_multicolumns/Projection_Input_3/calculate_gradf ==
  data: theta_hat input; gradf output; Theta_max input; epsilon input
function gradf = fcn(theta_hat,Theta_max, epsilon )
%#codegen
gradf = ( 2*(1+epsilon) ) / (epsilon*(Theta_max)^2) * theta_hat ;

== matlab function model_tmp_1p/Plant/Tether_Kite_Tether_UAV_Dynamics_1P/Tethermodel_Ground2Kite_1P/Tether_Ground2Kite ==
  data: x_dot input; x input; x_dotdot_TetherG2K output; v_w_vec input; d_tether parameter; CD_tether parameter; v_ro_set input; l_s input; c0 parameter; d0 parameter; rho_t parameter; g_vec parameter; rho_air parameter; l_tether output; l_s_dot output; xp_kite input; xp_dot_kite input
function [x_dotdot_TetherG2K,...
    l_tether, l_s_dot]    = fcn(x_dot, x,  v_w_vec,...
    d_tether, CD_tether, v_ro_set,l_s, c0, d0, rho_t, g_vec, rho_air, xp_kite, xp_dot_kite )

%#codegen
n = 10;
n_t_p = n-3;
l_tether = l_s * (n_t_p+1); % Tether length from ground to kite
l_s_dot = v_ro_set/(n_t_p+1);

% Adapt stiffness and damping with respect to current segment length
c = c0/l_s;
d = d0/l_s;

% Mass of tether segments with  respect to current segment length
m = l_s * rho_t;
m_vec = m * ones(n_t_p,1);

p_vec = x;
v_vec = x_dot;
p_norm = zeros(n_t_p,1);

% Vector with distances between particles
p_d = p_vec - [0;0;0; p_vec(1:3*n_t_p-3)];

% Vector with velocity differences
v_d = v_vec - [0;0;0; v_vec(1:3*n_t_p-3)];

% calculate absolute distances between points
for iter = 1 : n_t_p
    p_norm(iter) = norm( p_d( (iter-1)* 3 + 1 : (iter-1) * 3 + 3 ) );
end

%%------------------------------- Equations of motions-------------------------------
% Initialize matrices
fsd_tot_mat = zeros(3,n_t_p);
x_dotdot = zeros(3,n_t_p);
D_s_mat = zeros(3,n_t_p);

%% Set up equations of motions of ground to kite tether

% Boundary tether force from kite to particle below kite
f_kite = calcSpringDamperForce( c,norm( xp_kite - p_vec(3*(n-3) -2 : 3*(n-3) ) ), l_s, d,...
            xp_kite - p_vec(3*(n-3) -2 : 3*(n-3) ) ,...
            xp_dot_kite - v_vec(3*(n-3)), 1 );
        
for idx = 1 : n_t_p
    
    % Calculate Spring-Damper forces
    fsd_tot_mat(:,idx) = calcSpringDamperForce( c, p_norm(idx), l_s, d, p_d( (idx-1)*3+1:(idx-1)*3+3 ), v_d( (idx-1)*3+1:(idx-1)*3+3), idx );
    if idx < n_t_p
        fsd_tot_mat(:,idx+1) = calcSpringDamperForce( c, p_norm(idx+1), l_s, d, p_d( idx*3+1:idx*3+3 ), v_d( idx*3+1:idx*3+3), idx );       
    end
    
    % Calculate apparent wind speed of tether particles
    if idx == 1 % Segment that is connected to the ground
        v_a_p = v_w_vec - 0.5*x_dot(1:3) ;
    else
        v_a_p = v_w_vec - 0.5*( x_dot((idx-1)*3+1:(idx-1)*3+3) + x_dot((idx-1)*3:(idx-1)*3+2) ); % take mean value of adjacent particle vel. for segment velocity
    end
    
    % Calculate segment drag
    D_s_mat(:,idx) = calcSegmentDrag(p_d((idx-1)*3+1:(idx-1)*3+3) , v_a_p, rho_air, CD_tether, d_tether); % segment drag
    
    if idx < n_t_p
        % Equations of motion for the groud tether particles Newton x_dotdot = 1/m * (-f + u -mg )
        x_dotdot(:,idx) = 1/m_vec(idx) * ( -fsd_tot_mat(:,idx) + fsd_tot_mat(:,idx+1) - m_vec(idx)*g_vec  + D_s_mat(:,idx) );  % Particle dynamics
    else
        x_dotdot(:,idx) = 1/m_vec(idx) * ( -fsd_tot_mat(:,idx) + f_kite - m_vec(idx)*g_vec  + D_s_mat(:,idx) );  % Particle dynamics
    end
    
end


%% Reshape the structure of x_dotdot such that x_dotdot = [x1;y1;z1;x2;y2;...]
x_dotdot_TetherG2K = reshape(x_dotdot, [3*n_t_p,1]);

== matlab function model_tmp_1p/Plant/Tether_Kite_Tether_UAV_Dynamics_1P/Tethermodel_Kite2UAV/Tether_Kite2UAV ==
  data: launch_flag input; x_dotdot_p output; m_p parameter; g_vec parameter; xp_above input; xp input; xp_below input; xp_dot_above input; xp_dot input; xp_dot_below input; c0 parameter; d0 parameter; l_s0 parameter; CD_tether parameter; d_tether parameter; rho_air parameter; v_w_vec input
function x_dotdot_p = fcn(launch_flag, m_p, g_vec, xp_above, xp, xp_below, xp_dot_above, xp_dot, xp_dot_below,...
                        c0, d0, l_s0, CD_tether, d_tether, rho_air, v_w_vec  )
%#codegen
% Tether forces from below and above
f_T_below = calcSpringDamperForce(c0, norm(xp - xp_below) , l_s0, d0, xp - xp_below, xp_dot - xp_dot_below, 1 );
f_T_above = calcSpringDamperForce(c0, norm(xp_above - xp), l_s0, d0, xp_above - xp, xp_dot_above - xp_dot, 1 );

v_a_p = v_w_vec - 0.5 * ( xp_dot + xp_dot_above ) ; 
Dp = calcSegmentDrag( xp_above - xp  , v_a_p, rho_air, CD_tether, d_tether );

if launch_flag
    x_dotdot_p = 1/m_p * ( f_T_above - m_p*g_vec  + Dp ); % Particle dynamics
else
    x_dotdot_p = 1/m_p * ( -f_T_below + f_T_above - m_p*g_vec  + Dp );  %
end

== matlab function model_tmp_1p/Plant/Tether_Kite_Tether_UAV_Dynamics_1P/UAV_Model/Rotate thrust vector according to attitude ==
  data: u_Thrust_I input; eta input; u_Thrust_B output
function u_Thrust_B   = thrust_Bz_direction(  u_Thrust_I, eta) 

phi = eta(1); 
theta = eta(2); 
psi = eta(3); 

% Rotate thrust vector such that it is perpendicular to the "rotor blades"
u_Thrust_B = [cos(psi)*cos(theta), sin(psi)*cos(theta), -sin(theta); 
            cos(psi)*sin(theta)*sin(phi)-sin(psi)*cos(phi), sin(psi)*sin(theta)*sin(phi)+cos(psi)*cos(phi), cos(theta)*sin(phi); 
            cos(psi)*sin(theta)*cos(phi)+sin(psi)*sin(phi), sin(psi)*sin(theta)*cos(phi)-cos(psi)*sin(phi), cos(theta)*cos(phi)] *...
            [0;0;u_Thrust_I];

== matlab function model_tmp_1p/Plant/Tether_Kite_Tether_UAV_Dynamics_1P/UAV_Model/UAV_Dynamics ==
  data: x_dotdot_uav_trans output; omega_dot output; eta_dot output; Thrust input; m_uav parameter; g_vec parameter; x_UAV input; x_below_UAV input; x_dot_UAV input; x_dot_belowUAV input; c0 parameter; d0 parameter; l_s0 parameter; disturbance output; omega input; u_M input; J parameter; Jinv parameter; eta input
function [x_dotdot_uav_trans,omega_dot, eta_dot,  disturbance] = fcn(Thrust, m_uav, g_vec, x_UAV, x_below_UAV, x_dot_UAV, x_dot_belowUAV,...
    c0, d0, l_s0, omega, u_M, J,Jinv,eta )
%#codegen

%% Translational Dynamics
f_T_below = calcSpringDamperForce(c0, norm(x_UAV-x_below_UAV) , l_s0, d0, x_UAV-x_below_UAV, x_dot_UAV - x_dot_belowUAV, 1 );
disturbance = -f_T_below/m_uav;
%disturbance = 1/m_uav *[0;0;25] ;
x_dotdot_uav_trans = 1/m_uav * ( -1*f_T_below + Thrust - m_uav*g_vec + 0*[0;0;25]  ) ; % Drone dynamics

%% Rotational Dynamics 
p = omega(1); 
q = omega(2); 
r = omega(3); 
Ix = J(1,1); 
Iy = J(2,2); 
Iz = J(3,3); 

cross_coupling = [ Iy*q*r - Iz*q*r
                   Iz*p*r - Ix*p*r;
                   Ix*p*q - Iy*p*q];
% Bodyrate Dynamics
omega_dot = Jinv * ( cross_coupling + u_M ) ;  

% Attitude Dynamics
eta_dot = [1, sin(eta(1)) * tan(eta(2)), cos(eta(1)) * tan(eta(2)) ; 
0, cos(eta(1)), -sin(eta(1)); 
0, sin(eta(1))/cos(eta(2)), cos(eta(1))/cos(eta(2))] * omega ;

== matlab function model_tmp_1p/Controller/Inner_Loop_Attitude/Reference_Model1/Reference Model 2nd order ==
  data: eta_c input; eta_r_dot output; A_r input; B_r input; eta_r_dotdot output; x input
function [eta_r_dot, eta_r_dotdot] = fcn(eta_c, A_r, B_r, x)


x_dot = A_r * x + B_r * eta_c;

eta_r_dot = x_dot(1:3);
eta_r_dotdot = x_dot(4:6);

== matlab function model_tmp_1p/Flight_Path_Planner2/Reference_Dynamic_x1 ==
  data: x_cmd input; x_ref input; x_ref_dot output; t0 parameter; t1 parameter
function x_ref_dot = fcn(x_cmd, x_ref, t0, t1)

% a0 = 1;
% a1 = 5;

x_ref_dot = [0,1;
                -t0, -t1]*x_ref + [0;t0] * x_cmd;

== matlab function model_tmp_1p/Flight_Path_Planner2/Reference_Dynamic_x2 ==
  data: x_cmd input; x_ref input; x_ref_dot output; t0 parameter; t1 parameter
function x_ref_dot = fcn(x_cmd, x_ref, t0, t1)

% a0 = 1;
% a1 = 5;

x_ref_dot = [0,1;
                -t0, -t1]*x_ref + [0;t0] * x_cmd;
